simulink model "ckhsigselftestsigtest02"  (R2016a)
settings: Solver=VariableStepAuto  StartTime=0.0  StopTime=10.0  RelTol=1e-3
libraries: dspsrcs4 x1
settings Model: Creator=khung  LastModifiedBy=khung
settings DebuggingCC: SolverPrmCheckMsg=warning  AllowSymbolicDim=off
settings ModelReferenceCC: PropagateSignalLabelsOutOfModel=off
settings ConfigComp: CovModelRefEnable=Off  CovSFcnEnable=off

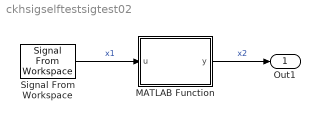
== system ckhsigselftestsigtest02 ==
  MATLAB Function : MATLAB Function  TreatAsAtomicUnit=on
  Signal From Workspace : dspsrcs4/Signal From Workspace  X=1:100  Ts=1  nsamps=1  OutputAfterFinalValue=Setting to zero  ignoreOrWarnInputAndFrameLengths=off  OutputFrames=off
  Out1 : Outport
  wires:
  Signal From Workspace/1 -> MATLAB Function/1(u)  "x1"
  MATLAB Function/1(y) -> Out1/1  "x2"

== matlab function ckhsigselftestsigtest02/MATLAB Function ==
  data: u input; y output
function y = fcn(u)
%#codegen

y = u;
% size(y)
